simulink model "Quadrotor"  (R2022b)
settings: Solver=FixedStepAuto  StartTime=0.0  StopTime=1000  FixedStep=0.0005  RelTol=1e-3
model workspace (MAT data in the model file):
  b = 0.000142
  g = 9.8
  m = 1
undefined symbols (not defined in the file): Pitch, Roll, X, Y, Yaw, Z
libraries: simulink x12, slpidlib x9, sharedtransform x1, uavutilslib x1, aerolibanim x1
(part 1 of 3)
settings Model: Creator=huawei  LastModifiedBy=Powehi
settings SolverCC: ZeroCrossAlgorithm=Adaptive
settings DebuggingCC: IgnoredZcDiagnostic=none  UnconnectedInputMsg=warning  UnconnectedOutputMsg=warning  UnconnectedLineMsg=warning  SFMachineParentedDataDiag=warning
settings ModelReferenceCC: EnableRefExpFcnMdlSchedulingChecks=on

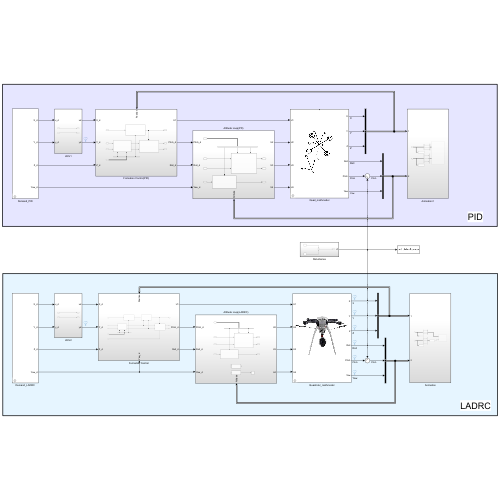
[thumbnail: Simulink's stored preview of the top-level diagram]
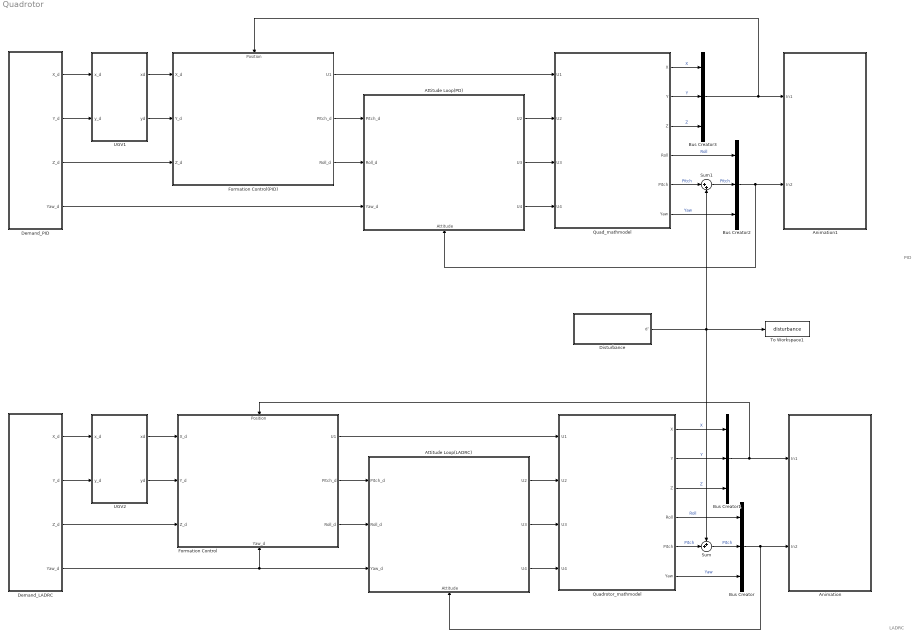
== system Quadrotor ==
  note: PID
  note: LADRC
  Animation : Subsystem
  Animation1 : Subsystem
  Attitude Loop(LADRC) : Subsystem
      settings: PortSchema="{\"entries\":[{\"content\":{\"sides\":[{\"content\":{\"connectorIds\":[\"In1\",\"In2\",\"In3\"]},\"type\":\"ConnectorPlacement.EquallySpacedRectSide\",\"uuid\":\"741c63cb-3193-49ed-b6fe-0554dd8eb38b\"},{\"content\":{\"connectorIds\":[\"Out1\",\"Out2\",\"Out3\"],\"side\":\"RIGHT\"},\"type\":\"ConnectorPlacement.EquallySpacedRectSide\",\"uuid\":\"55d4e1d6-ced0-4d00-88f3-94ecae3eab08\"},{\"content\":{\"connectorIds\":[],\"side\":\"TOP\"},\"type\":\"ConnectorPlacement.EquallySpacedRectSide\",\"uuid\":\"670d5dfa-1a50-4aee-963c-097076b25aa9\"},{\"content\":{\"connectorIds\":[\"In4\"],\"side\":\"BOTTOM\"},\"type\":\"ConnectorPlacement.EquallySpacedRectSide\",\"uuid\":\"461487f9-9010-46f7-8d40-b6bfcadca1df\"}]},\"type\":\"ConnectorPlacement.EquallySpacedConnector\",\"uuid\":\"b0fd4550-2f46-4562-9b6e-a30bcd34312f\"}],\"packageUris\":[\"http://schema.mathworks.com/mf0/Connector/19700101\"],\"version\":\"1.0\"}"
  Attitude Loop(PD) : Subsystem
      settings: PortSchema="{\"entries\":[{\"content\":{\"sides\":[{\"content\":{\"connectorIds\":[\"In1\",\"In2\",\"In3\"]},\"type\":\"ConnectorPlacement.EquallySpacedRectSide\",\"uuid\":\"741c63cb-3193-49ed-b6fe-0554dd8eb38b\"},{\"content\":{\"connectorIds\":[\"Out1\",\"Out2\",\"Out3\"],\"side\":\"RIGHT\"},\"type\":\"ConnectorPlacement.EquallySpacedRectSide\",\"uuid\":\"55d4e1d6-ced0-4d00-88f3-94ecae3eab08\"},{\"content\":{\"connectorIds\":[],\"side\":\"TOP\"},\"type\":\"ConnectorPlacement.EquallySpacedRectSide\",\"uuid\":\"670d5dfa-1a50-4aee-963c-097076b25aa9\"},{\"content\":{\"connectorIds\":[\"In4\"],\"side\":\"BOTTOM\"},\"type\":\"ConnectorPlacement.EquallySpacedRectSide\",\"uuid\":\"461487f9-9010-46f7-8d40-b6bfcadca1df\"}]},\"type\":\"ConnectorPlacement.EquallySpacedConnector\",\"uuid\":\"b0fd4550-2f46-4562-9b6e-a30bcd34312f\"}],\"packageUris\":[\"http://schema.mathworks.com/mf0/Connector/R2020b\"],\"version\":\"1.0\"}"
  Bus Creator : BusCreator  Inputs=Roll,Pitch,Yaw
  Bus Creator1 : BusCreator  Inputs=X,Y,Z
  Bus Creator2 : BusCreator  Inputs=Roll,Pitch,Yaw
  Bus Creator3 : BusCreator  Inputs=X,Y,Z
  Demand_LADRC : Subsystem  mask{s=4}
      mask DialogControl ParameterGroupVar Prompt: 轨迹选择
      mask DialogControl Control8 Prompt: 请输入轨迹序号
      mask DialogControl Container7 Prompt: 展开
      mask DialogControl Control1 Prompt: 1.上升
      mask DialogControl Control2 Prompt: 2.直线
      mask DialogControl Control3 Prompt: 3.环形轨迹
      mask DialogControl Control4 Prompt: 4.螺旋轨迹
      mask DialogControl Control5 Prompt: 5.蝶形轨迹
      mask DialogControl Control7 Prompt: 启动
      mask DialogControl Control7 Callback:
      | clear
      | sim('Quadrotor')
      | figure(1)
      | 
      |   comet3(ans.position(:,1),ans.position(:,2),ans.position(:,end),0.1)%彗星/动图轨迹
      |   title('飞行动态显示图')
      |   grid on
      | 
      | figure(2)
      | subplot(2,2,1)%轨迹线图
      |   plot3(ans.position(:,1),ans.position(:,2),ans.position(:,end),"r",'LineWidth',2) ;%绘制轨迹线图
      |    hold on
      |   plot3(ans.demand(:,1),ans.demand(:,2),ans.demand(:,3),"b--",'LineWidth',2) %绘制输入
      |    hold on
      |    plot3(0,0,0,'g.','markersize',30)%标起始位置
      |    xlabel('X/m');ylabel('Y/m');zlabel('Z/m');%坐标轴名称
      |    legend('飞行轨迹','给定路线')
      |    text(0,0,0,'起始点')
      |    title('飞行轨迹图')
      |    grid on
      | 
      | subplot(2,2,2)%x跟踪对比
      | 
      |    plot(ans.position(:,1),'r','LineWidth',2)%x输出
      |     hold on
      |    plot(ans.demand(:,1),'b--','LineWidth',2)%x给定值
      |     set(gca,'XTick',0:400000:2000000);set(gca,'XTicklabel',{'0','200','400','600','800','1000'})%标定刻度
      |     xlabel('t/s');ylabel('X&Xd');%坐标轴名称
      |     axis([0 inf -1.5 1.5])%坐标范围
      |     legend('x','xd')
      |     title('X坐标跟踪')
      |     grid on%网格
      | 
      | subplot(2,2,3)%y跟踪对比
      | 
      |    plot(ans.position(:,2),'r','LineWidth',2)
      |     hold on
      |    plot(ans.demand(:,2),'b--','LineWidth',2)
      |     set(gca,'XTick',0:400000:2000000);set(gca,'XTicklabel',{'0','200','400','600','800','1000'})
      |     xlabel('t/s');ylabel('Y&Yd');
      |     axis([0 inf -1.5 1.5])
      |     legend('y','yd')
      |     title('Y坐标跟踪')
      |     grid on
      | subplot(2,2,4)%z跟踪对比
      | 
      |    plot(ans.position(:,end),'r','LineWidth',2)
      |     hold on
      |    plot(ans.demand(:,3),'b--','LineWidth',2)
      |     set(gca,'XTick',0:400000:2000000);set(gca,'XTicklabel',{'0','200','400','600','800','1000'})
      |     xlabel('t/s');ylabel('Z&Zd');
      |     axis([0 inf 0 7])
      |     legend('z','zd')
      |     title('Z坐标跟踪')
      |     grid on
  Demand_PID : Subsystem  mask{s=4}
      mask DialogControl ParameterGroupVar Prompt: 轨迹选择
      mask DialogControl Control8 Prompt: 请输入轨迹序号
      mask DialogControl Container7 Prompt: 展开
      mask DialogControl Control1 Prompt: 1.上升
      mask DialogControl Control2 Prompt: 2.直线
      mask DialogControl Control3 Prompt: 3.环形轨迹
      mask DialogControl Control4 Prompt: 4.螺旋轨迹
      mask DialogControl Control5 Prompt: 5.蝶形轨迹
      mask DialogControl Control7 Prompt: 启动
      mask DialogControl Control7 Callback:
      | clear
      | sim('Quadrotor_PID_final')
      | figure(1)
      | 
      |   comet3(ans.position(:,1),ans.position(:,2),ans.position(:,end),0.1)%彗星/动图轨迹
      |   title('飞行动态显示图')
      |   grid on
      | 
      | figure(2)
      | subplot(2,2,1)%轨迹线图
      |   plot3(ans.position(:,1),ans.position(:,2),ans.position(:,end),"r",'LineWidth',2) ;%绘制轨迹线图
      |    hold on
      |   plot3(ans.demand(:,1),ans.demand(:,2),ans.demand(:,3),"b--",'LineWidth',2) %绘制输入
      |    hold on
      |    plot3(0,0,0,'g.','markersize',30)%标起始位置
      |    xlabel('X/m');ylabel('Y/m');zlabel('Z/m');%坐标轴名称
      |    legend('飞行轨迹','给定路线')
      |    text(0,0,0,'起始点')
      |    title('飞行轨迹图')
      |    grid on
      | 
      | subplot(2,2,2)%x跟踪对比
      | 
      |    plot(ans.position(:,1),'r','LineWidth',2)%x输出
      |     hold on
      |    plot(ans.demand(:,1),'b--','LineWidth',2)%x给定值
      |     set(gca,'XTick',0:1200:6000);set(gca,'XTicklabel',{'0','200','400','600','800','1000'})%标定刻度
      |     xlabel('t/s');ylabel('X&Xd');%坐标轴名称
      |     axis([0 inf -1.5 1.5])%坐标范围
      |     legend('x','xd')
      |     title('X坐标跟踪')
      |     grid on%网格
      | 
      | subplot(2,2,3)%y跟踪对比
      | 
      |    plot(ans.position(:,2),'r','LineWidth',2)
      |     hold on
      |    plot(ans.demand(:,2),'b--','LineWidth',2)
      |     set(gca,'XTick',0:1200:6000);set(gca,'XTicklabel',{'0','200','400','600','800','1000'})
      |     xlabel('t/s');ylabel('Y&Yd');
      |     axis([0 inf -1.5 1.5])
      |     legend('y','yd')
      |     title('Y坐标跟踪')
      |     grid on
      | subplot(2,2,4)%z跟踪对比
      | 
      |    plot(ans.position(:,end),'r','LineWidth',2)
      |     hold on
      |    plot(ans.demand(:,3),'b--','LineWidth',2)
      |     set(gca,'XTick',0:1200:6000);set(gca,'XTicklabel',{'0','200','400','600','800','1000'})
      |     xlabel('t/s');ylabel('Z&Zd');
      |     axis([0 inf 0 7])
      |     legend('z','zd')
      |     title('Z坐标跟踪')
      |     grid on
  Disturbance : Subsystem
  Formation Control : Subsystem
      settings: PortSchema="{\"entries\":[{\"content\":{\"sides\":[{\"content\":{\"connectorIds\":[\"In1\",\"In2\",\"In3\"]},\"type\":\"ConnectorPlacement.EquallySpacedRectSide\",\"uuid\":\"741c63cb-3193-49ed-b6fe-0554dd8eb38b\"},{\"content\":{\"connectorIds\":[\"Out1\",\"Out2\",\"Out3\"],\"side\":\"RIGHT\"},\"type\":\"ConnectorPlacement.EquallySpacedRectSide\",\"uuid\":\"55d4e1d6-ced0-4d00-88f3-94ecae3eab08\"},{\"content\":{\"connectorIds\":[\"In4\"],\"side\":\"TOP\"},\"type\":\"ConnectorPlacement.EquallySpacedRectSide\",\"uuid\":\"670d5dfa-1a50-4aee-963c-097076b25aa9\"},{\"content\":{\"connectorIds\":[\"In5\"],\"side\":\"BOTTOM\"},\"type\":\"ConnectorPlacement.EquallySpacedRectSide\",\"uuid\":\"31dc6e32-e4ae-4a63-8318-e80959689dd0\"}]},\"type\":\"ConnectorPlacement.EquallySpacedConnector\",\"uuid\":\"b0fd4550-2f46-4562-9b6e-a30bcd34312f\"}],\"packageUris\":[\"http://schema.mathworks.com/mf0/Connector/R2020b\"],\"version\":\"1.0\"}"
  Formation Control(PID) : Subsystem
      settings: PortSchema="{\"entries\":[{\"content\":{\"sides\":[{\"content\":{\"connectorIds\":[\"In1\",\"In2\",\"In3\"]},\"type\":\"ConnectorPlacement.EquallySpacedRectSide\",\"uuid\":\"741c63cb-3193-49ed-b6fe-0554dd8eb38b\"},{\"content\":{\"connectorIds\":[\"Out1\",\"Out2\",\"Out3\"],\"side\":\"RIGHT\"},\"type\":\"ConnectorPlacement.EquallySpacedRectSide\",\"uuid\":\"55d4e1d6-ced0-4d00-88f3-94ecae3eab08\"},{\"content\":{\"connectorIds\":[\"In4\"],\"side\":\"TOP\"},\"type\":\"ConnectorPlacement.EquallySpacedRectSide\",\"uuid\":\"670d5dfa-1a50-4aee-963c-097076b25aa9\"},{\"content\":{\"connectorIds\":[],\"side\":\"BOTTOM\"},\"type\":\"ConnectorPlacement.EquallySpacedRectSide\",\"uuid\":\"31dc6e32-e4ae-4a63-8318-e80959689dd0\"}]},\"type\":\"ConnectorPlacement.EquallySpacedConnector\",\"uuid\":\"b0fd4550-2f46-4562-9b6e-a30bcd34312f\"}],\"packageUris\":[\"http://schema.mathworks.com/mf0/Connector/R2020b\"],\"version\":\"1.0\"}"
  Quad_mathmodel : Subsystem  mask{m=1, L=0.24, b=1.42e-4, d=6.21e-5, g=9.8, Ix=8.1e-3, Iy=8.1e-3, Iz=12.4e-3, Jtp=7.24e-5}
      mask DialogControl ParameterGroupVar Prompt: 四旋翼飞行器参数设置
      mask DialogControl Container10 Prompt: 飞行器质量(kg)
      mask DialogControl Container11 Prompt: 质心到电机中心轴距(m)
      mask DialogControl Container16 Prompt: 升力系数
      mask DialogControl Container15 Prompt: 阻力系数
      mask DialogControl Container14 Prompt: 重力加速度
      mask DialogControl Container13 Prompt: 绕X轴转动惯量
      mask DialogControl Container12 Prompt: 绕Y轴转动惯量
      mask DialogControl Container17 Prompt: 绕Z轴转动惯量
      mask DialogControl Container18 Prompt: 机体绕转轴的总转动惯量（可忽略）
      mask Display: image('$imagefile'); % Use "Edit Image" on toolstrip to change.
  Quadrotor_mathmodel : Subsystem  mask{m=1, L=0.24, b=1.42e-4, d=6.21e-5, g=9.8, Ix=8.1e-3, Iy=8.1e-3, Iz=12.4e-3, Jtp=7.24e-5}
      mask DialogControl ParameterGroupVar Prompt: 四旋翼飞行器参数设置
      mask DialogControl Container10 Prompt: 飞行器质量(kg)
      mask DialogControl Container11 Prompt: 质心到电机中心轴距(m)
      mask DialogControl Container16 Prompt: 升力系数
      mask DialogControl Container15 Prompt: 阻力系数
      mask DialogControl Container14 Prompt: 重力加速度
      mask DialogControl Container13 Prompt: 绕X轴转动惯量
      mask DialogControl Container12 Prompt: 绕Y轴转动惯量
      mask DialogControl Container17 Prompt: 绕Z轴转动惯量
      mask DialogControl Container18 Prompt: 机体绕转轴的总转动惯量（可忽略）
      mask Display: image('$imagefile'); % Use "Edit Image" on toolstrip to change.
  Sum : Sum  Inputs=++|
  Sum1 : Sum  Inputs=|++
  To Workspace1 : ToWorkspace  VariableName=disturbance  SampleTime=-1
  UGV1 : Subsystem
  UGV2 : Subsystem
  wires:
  Quadrotor_mathmodel/6(Yaw) -> Bus Creator/3  "Yaw"
  Quadrotor_mathmodel/3(Z) -> Bus Creator1/3  "Z"
  Formation Control/1(U1) -> Quadrotor_mathmodel/1(U1)
  Formation Control/2(Pitch_d) -> Attitude Loop(LADRC)/1(Pitch_d)
  Formation Control/3(Roll_d) -> Attitude Loop(LADRC)/2(Roll_d)
  Attitude Loop(LADRC)/3(U4) -> Quadrotor_mathmodel/4(U4)
  Attitude Loop(LADRC)/1(U2) -> Quadrotor_mathmodel/2(U2)
  Attitude Loop(LADRC)/2(U3) -> Quadrotor_mathmodel/3(U3)
  Quadrotor_mathmodel/4(Roll) -> Bus Creator/1  "Roll"
  Bus Creator1/1 -> Animation/1(In1), Formation Control/4(Position)
  Bus Creator/1 -> Attitude Loop(LADRC)/4(Attitude), Animation/2(In2)
  Demand_LADRC/1(X_d) -> UGV2/1(x_d)
  UGV2/1(xd) -> Formation Control/1(X_d)
  Demand_LADRC/2(Y_d) -> UGV2/2(y_d)
  UGV2/2(yd) -> Formation Control/2(Y_d)
  Demand_LADRC/3(Z_d) -> Formation Control/3(Z_d)
  Demand_LADRC/4(Yaw_d) -> Formation Control/5(Yaw_d), Attitude Loop(LADRC)/3(Yaw_d)
  Quadrotor_mathmodel/1(X) -> Bus Creator1/1  "X"
  Quadrotor_mathmodel/2(Y) -> Bus Creator1/2  "Y"
  Sum/1 -> Bus Creator/2  "Pitch"
  Quadrotor_mathmodel/5(Pitch) -> Sum/2  "Pitch"
  Disturbance/1(d') -> To Workspace1/1, Sum1/2, Sum/1
  Demand_PID/3(Z_d) -> Formation Control(PID)/3(Z_d)
  Quad_mathmodel/1(X) -> Bus Creator3/1  "X"
  Demand_PID/4(Yaw_d) -> Attitude Loop(PD)/3(Yaw_d)
  Attitude Loop(PD)/1(U2) -> Quad_mathmodel/2(U2)
  Quad_mathmodel/3(Z) -> Bus Creator3/3  "Z"
  Attitude Loop(PD)/3(U4) -> Quad_mathmodel/4(U4)
  Attitude Loop(PD)/2(U3) -> Quad_mathmodel/3(U3)
  Formation Control(PID)/3(Roll_d) -> Attitude Loop(PD)/2(Roll_d)
  Bus Creator2/1 -> Attitude Loop(PD)/4(Attitude), Animation1/2(In2)
  Quad_mathmodel/2(Y) -> Bus Creator3/2  "Y"
  Quad_mathmodel/4(Roll) -> Bus Creator2/1  "Roll"
  Formation Control(PID)/2(Pitch_d) -> Attitude Loop(PD)/1(Pitch_d)
  Formation Control(PID)/1(U1) -> Quad_mathmodel/1(U1)
  Bus Creator3/1 -> Formation Control(PID)/4(Position), Animation1/1(In1)
  Quad_mathmodel/6(Yaw) -> Bus Creator2/3  "Yaw"
  Sum1/1 -> Bus Creator2/2  "Pitch"
  Quad_mathmodel/5(Pitch) -> Sum1/1  "Pitch"
  UGV1/1(xd) -> Formation Control(PID)/1(X_d)
  UGV1/2(yd) -> Formation Control(PID)/2(Y_d)
  Demand_PID/2(Y_d) -> UGV1/2(y_d)
  Demand_PID/1(X_d) -> UGV1/1(x_d)

== system Quadrotor/Animation ==
  In1 : Inport
  In2 : Inport  Port=2
  Bus Creator2 : BusCreator  Inputs=3
  Bus Creator3 : BusCreator  Inputs=3
  Bus Selector : BusSelector  OutputSignals=X,Y,Z
  Bus Selector1 : BusSelector  OutputSignals=Roll,Pitch,Yaw
  Rotation Angles to Quaternions : sharedtransform/Rotation Angles to Quaternions  rotationOrder=XYZ  aMode=aMode
  To Workspace : ToWorkspace  VariableName=position1  SampleTime=-1
  To Workspace1 : ToWorkspace  VariableName=attitude1  SampleTime=-1
  UAV Animation : uavutilslib/UAV Animation  Commented=on  UAVType=Multirotor  UAVSize=0.1  InertialZDirection=Up  SampleTime=-1
  wires:
  In1/1 -> Bus Selector/1, To Workspace/1
  Bus Selector1/1 -> Bus Creator2/1  "<Roll>"
  In2/1 -> To Workspace1/1, Bus Selector1/1
  Bus Selector/2 -> Bus Creator3/2  "<Y>"
  Bus Selector1/2 -> Bus Creator2/2  "<Pitch>"
  Bus Selector/3 -> Bus Creator3/3  "<Z>"
  Bus Selector/1 -> Bus Creator3/1  "<X>"
  Bus Selector1/3 -> Bus Creator2/3  "<Yaw>"
  Bus Creator2/1 -> Rotation Angles to Quaternions/1
  Rotation Angles to Quaternions/1 -> UAV Animation/2
  Bus Creator3/1 -> UAV Animation/1

== system Quadrotor/Animation1 ==
  In1 : Inport
  In2 : Inport  Port=2
  6DoF Animation : aerolibanim/6DoF Animation  Commented=on  u1=[-2 2 -2 2 -4 0]  u2=0.1  u3=0.5  u4=[0 0 4]  u5=Fixed position  u6=[40 0 -0.5]  u7=7  u8=on
  Bus Creator2 : BusCreator  Inputs=3
  Bus Creator3 : BusCreator  Inputs=3
  Bus Selector : BusSelector  OutputSignals=X,Y,Z
  Bus Selector1 : BusSelector  OutputSignals=Roll,Pitch,Yaw
  To Workspace : ToWorkspace  VariableName=position  SampleTime=-1
  To Workspace1 : ToWorkspace  VariableName=attitude  SampleTime=-1
  wires:
  In1/1 -> Bus Selector/1, To Workspace/1
  Bus Selector1/1 -> Bus Creator2/1  "<Roll>"
  In2/1 -> To Workspace1/1, Bus Selector1/1
  Bus Selector/2 -> Bus Creator3/2  "<Y>"
  Bus Selector1/2 -> Bus Creator2/2  "<Pitch>"
  Bus Creator2/1 -> 6DoF Animation/2
  Bus Selector/3 -> Bus Creator3/3  "<Z>"
  Bus Creator3/1 -> 6DoF Animation/1
  Bus Selector/1 -> Bus Creator3/1  "<X>"
  Bus Selector1/3 -> Bus Creator2/3  "<Yaw>"

== system Quadrotor/Attitude Loop(LADRC) ==
  Pitch_d : Inport
  Roll_d : Inport  Port=2
  Yaw_d : Inport  Port=3
  Attitude : Inport  Port=4
  Bus Selector : BusSelector  OutputSignals=Yaw,Pitch,Roll
  LADRC : Subsystem  mask{h=0.0005, r=100, beta01=100, beta02=200, beta03=300, kp1=5, kp2=5, b=1}
      mask DialogControl ParameterGroupVar Prompt: 四旋翼参数
      mask DialogControl Container3 Prompt: 步长
      mask DialogControl Container4 Prompt: 跟踪速度
      mask DialogControl Container5 Prompt: 增益
      mask DialogControl Container6 Prompt: 系统增益
  LADRC1 : Subsystem  mask{h=0.0005, r=100, beta01=100, beta02=200, beta03=300, kp1=5, kp2=5, b=1}
      mask DialogControl ParameterGroupVar Prompt: 四旋翼参数
      mask DialogControl Container3 Prompt: 步长
      mask DialogControl Container4 Prompt: 跟踪速度
      mask DialogControl Container5 Prompt: 增益
      mask DialogControl Container6 Prompt: 系统增益
  P&R : Subsystem
      settings: PortSchema="{\"entries\":[{\"content\":{\"sides\":[{\"content\":{\"connectorIds\":[\"In1\",\"In2\"]},\"type\":\"ConnectorPlacement.EquallySpacedRectSide\",\"uuid\":\"5a168f57-9082-4ef9-b723-ec42d235f15b\"},{\"content\":{\"connectorIds\":[\"Out1\",\"Out2\"],\"side\":\"RIGHT\"},\"type\":\"ConnectorPlacement.EquallySpacedRectSide\",\"uuid\":\"1b4dc671-5a32-4537-87d8-64b7817d412d\"},{\"content\":{\"connectorIds\":[\"In3\",\"In4\"],\"side\":\"TOP\"},\"type\":\"ConnectorPlacement.EquallySpacedRectSide\",\"uuid\":\"3d489923-4a97-462b-9fd9-288b2bf2a159\"}]},\"type\":\"ConnectorPlacement.EquallySpacedConnector\",\"uuid\":\"91228c47-fce9-4c1d-8a3a-204dc80f90dd\"}],\"packageUris\":[\"http://schema.mathworks.com/mf0/Connector/R2020b\"],\"version\":\"1.0\"}"
  Scope : Scope
  yaw : Subsystem
      settings: PortSchema="{\"entries\":[{\"content\":{\"sides\":[{\"content\":{\"connectorIds\":[\"In1\"]},\"type\":\"ConnectorPlacement.EquallySpacedRectSide\",\"uuid\":\"a7b1533a-1266-40d5-b52c-012082b26468\"},{\"content\":{\"connectorIds\":[\"Out1\"],\"side\":\"RIGHT\"},\"type\":\"ConnectorPlacement.EquallySpacedRectSide\",\"uuid\":\"b4620233-0e85-40ae-9738-c29ba1209ef5\"},{\"content\":{\"connectorIds\":[\"In2\"],\"side\":\"TOP\"},\"type\":\"ConnectorPlacement.EquallySpacedRectSide\",\"uuid\":\"ab9c222c-25de-47f6-b54f-342fd8d0321b\"},{\"content\":{\"connectorIds\":[],\"side\":\"BOTTOM\"},\"type\":\"ConnectorPlacement.EquallySpacedRectSide\",\"uuid\":\"5eacbb93-3d5d-4d57-aaef-fda87c8b1f96\"}]},\"type\":\"ConnectorPlacement.EquallySpacedConnector\",\"uuid\":\"8cc1c8e9-c992-4e05-8575-ab9d3ec9e6a4\"}],\"packageUris\":[\"http://schema.mathworks.com/mf0/Connector/R2020b\"],\"version\":\"1.0\"}"
  U2 : Outport
  U3 : Outport  Port=2
  U4 : Outport  Port=3
  wires:
  Bus Selector/2 -> P&R/3(Pitch)  "<Pitch>"
  Roll_d/1 -> P&R/2(Roll_d)
  yaw/1(U4) -> U4/1
  Attitude/1 -> Bus Selector/1
  Bus Selector/3 -> P&R/4(Roll)  "<Roll>"
  Pitch_d/1 -> P&R/1(Pitch_d)
  Bus Selector/1 -> yaw/2(Yaw)  "<Yaw>"
  P&R/2(U2) -> U2/1
  P&R/1(U3) -> U3/1
  Yaw_d/1 -> yaw/1(Yaw_d)
  LADRC/1(y) -> Scope/1

== system Quadrotor/Attitude Loop(PD) ==
  Pitch_d : Inport
  Roll_d : Inport  Port=2
  Yaw_d : Inport  Port=3
  Attitude : Inport  Port=4
  Bus Selector : BusSelector  OutputSignals=Yaw,Pitch,Roll
  P&R : Subsystem
      settings: PortSchema="{\"entries\":[{\"content\":{\"sides\":[{\"content\":{\"connectorIds\":[\"In1\",\"In2\"]},\"type\":\"ConnectorPlacement.EquallySpacedRectSide\",\"uuid\":\"5a168f57-9082-4ef9-b723-ec42d235f15b\"},{\"content\":{\"connectorIds\":[\"Out1\",\"Out2\"],\"side\":\"RIGHT\"},\"type\":\"ConnectorPlacement.EquallySpacedRectSide\",\"uuid\":\"1b4dc671-5a32-4537-87d8-64b7817d412d\"},{\"content\":{\"connectorIds\":[\"In3\",\"In4\"],\"side\":\"TOP\"},\"type\":\"ConnectorPlacement.EquallySpacedRectSide\",\"uuid\":\"3d489923-4a97-462b-9fd9-288b2bf2a159\"}]},\"type\":\"ConnectorPlacement.EquallySpacedConnector\",\"uuid\":\"91228c47-fce9-4c1d-8a3a-204dc80f90dd\"}],\"packageUris\":[\"http://schema.mathworks.com/mf0/Connector/R2020b\"],\"version\":\"1.0\"}"
  yaw : Subsystem
      settings: PortSchema="{\"entries\":[{\"content\":{\"sides\":[{\"content\":{\"connectorIds\":[\"In1\"]},\"type\":\"ConnectorPlacement.EquallySpacedRectSide\",\"uuid\":\"a7b1533a-1266-40d5-b52c-012082b26468\"},{\"content\":{\"connectorIds\":[\"Out1\"],\"side\":\"RIGHT\"},\"type\":\"ConnectorPlacement.EquallySpacedRectSide\",\"uuid\":\"b4620233-0e85-40ae-9738-c29ba1209ef5\"},{\"content\":{\"connectorIds\":[\"In2\"],\"side\":\"TOP\"},\"type\":\"ConnectorPlacement.EquallySpacedRectSide\",\"uuid\":\"ab9c222c-25de-47f6-b54f-342fd8d0321b\"},{\"content\":{\"connectorIds\":[],\"side\":\"BOTTOM\"},\"type\":\"ConnectorPlacement.EquallySpacedRectSide\",\"uuid\":\"5eacbb93-3d5d-4d57-aaef-fda87c8b1f96\"}]},\"type\":\"ConnectorPlacement.EquallySpacedConnector\",\"uuid\":\"8cc1c8e9-c992-4e05-8575-ab9d3ec9e6a4\"}],\"packageUris\":[\"http://schema.mathworks.com/mf0/Connector/R2020b\"],\"version\":\"1.0\"}"
  U2 : Outport
  U3 : Outport  Port=2
  U4 : Outport  Port=3
  wires:
  Bus Selector/2 -> P&R/3(Pitch)  "<Pitch>"
  Roll_d/1 -> P&R/2(Roll_d)
  yaw/1(U4) -> U4/1
  Attitude/1 -> Bus Selector/1
  Bus Selector/3 -> P&R/4(Roll)  "<Roll>"
  Pitch_d/1 -> P&R/1(Pitch_d)
  Bus Selector/1 -> yaw/2(Yaw)  "<Yaw>"
  P&R/2(U2) -> U2/1
  P&R/1(U3) -> U3/1
  Yaw_d/1 -> yaw/1(Yaw_d)

== system Quadrotor/Demand_LADRC ==
  Multiport Switch : MultiPortSwitch  Inputs=6  SaturateOnIntegerOverflow=off  InputSameDT=off
  generate : Subsystem
  out : Subsystem
  select number : Constant  Value=s
  X_d : Outport
  Y_d : Outport  Port=2
  Z_d : Outport  Port=3
  Yaw_d : Outport  Port=4
  wires:
  out/1(X_d) -> X_d/1
  out/2(Y_d) -> Y_d/1
  out/3(Z_d) -> Z_d/1
  out/4(Yaw_d) -> Yaw_d/1
  Multiport Switch/1 -> out/1(In1)
  generate/1(up) -> Multiport Switch/2
  generate/2(ramp) -> Multiport Switch/3
  generate/3(circle) -> Multiport Switch/4
  generate/4(screw) -> Multiport Switch/5
  generate/5(butterfiy) -> Multiport Switch/6
  select number/1 -> Multiport Switch/1
  generate/6(steady) -> Multiport Switch/7

== system Quadrotor/Demand_PID ==
  Multiport Switch : MultiPortSwitch  Inputs=6  SaturateOnIntegerOverflow=off  InputSameDT=off
  generate : Subsystem
  out : Subsystem
  select number : Constant  Value=s
  X_d : Outport
  Y_d : Outport  Port=2
  Z_d : Outport  Port=3
  Yaw_d : Outport  Port=4
  wires:
  out/1(X_d) -> X_d/1
  out/2(Y_d) -> Y_d/1
  out/3(Z_d) -> Z_d/1
  out/4(Yaw_d) -> Yaw_d/1
  Multiport Switch/1 -> out/1(In1)
  generate/1(up) -> Multiport Switch/2
  generate/2(ramp) -> Multiport Switch/3
  generate/3(circle) -> Multiport Switch/4
  generate/4(screw) -> Multiport Switch/5
  generate/5(butterfiy) -> Multiport Switch/6
  select number/1 -> Multiport Switch/1
  generate/6(steady) -> Multiport Switch/7

== system Quadrotor/Disturbance ==
  Step : Step  Time=20  After=0.01  SampleTime=0.0005
  Step1 : Step  Time=22  After=-0.01  SampleTime=0.0005
  Sum : Sum
  d' : Outport
  wires:
  Step/1 -> Sum/1
  Step1/1 -> Sum/2
  Sum/1 -> d'/1

== system Quadrotor/Formation Control ==
  X_d : Inport
  Y_d : Inport  Port=2
  Z_d : Inport  Port=3
  Position : Inport  Port=4
  Yaw_d : Inport  Port=5
  Bus Selector1 : BusSelector  OutputSignals=X,Y,Z
  height : Subsystem
      settings: PortSchema="{\"entries\":[{\"content\":{\"sides\":[{\"content\":{\"connectorIds\":[\"In1\"]},\"type\":\"ConnectorPlacement.EquallySpacedRectSide\",\"uuid\":\"a7b1533a-1266-40d5-b52c-012082b26468\"},{\"content\":{\"connectorIds\":[\"Out1\"],\"side\":\"RIGHT\"},\"type\":\"ConnectorPlacement.EquallySpacedRectSide\",\"uuid\":\"b4620233-0e85-40ae-9738-c29ba1209ef5\"},{\"content\":{\"connectorIds\":[],\"side\":\"TOP\"},\"type\":\"ConnectorPlacement.EquallySpacedRectSide\",\"uuid\":\"ab9c222c-25de-47f6-b54f-342fd8d0321b\"},{\"content\":{\"connectorIds\":[\"In2\"],\"side\":\"BOTTOM\"},\"type\":\"ConnectorPlacement.EquallySpacedRectSide\",\"uuid\":\"c0ec5864-a2e3-4dc9-86df-2e8e31dc698f\"}]},\"type\":\"ConnectorPlacement.EquallySpacedConnector\",\"uuid\":\"8cc1c8e9-c992-4e05-8575-ab9d3ec9e6a4\"}],\"packageUris\":[\"http://schema.mathworks.com/mf0/Connector/R2020b\"],\"version\":\"1.0\"}"
  "location " : Subsystem
      settings: PortSchema="{\"entries\":[{\"content\":{\"sides\":[{\"content\":{\"connectorIds\":[\"In1\",\"In2\"]},\"type\":\"ConnectorPlacement.EquallySpacedRectSide\",\"uuid\":\"5a168f57-9082-4ef9-b723-ec42d235f15b\"},{\"content\":{\"connectorIds\":[\"Out1\",\"Out2\"],\"side\":\"RIGHT\"},\"type\":\"ConnectorPlacement.EquallySpacedRectSide\",\"uuid\":\"1b4dc671-5a32-4537-87d8-64b7817d412d\"},{\"content\":{\"connectorIds\":[],\"side\":\"TOP\"},\"type\":\"ConnectorPlacement.EquallySpacedRectSide\",\"uuid\":\"3d489923-4a97-462b-9fd9-288b2bf2a159\"},{\"content\":{\"connectorIds\":[\"In3\",\"In4\"],\"side\":\"BOTTOM\"},\"type\":\"ConnectorPlacement.EquallySpacedRectSide\",\"uuid\":\"ca455ebd-18aa-4cdd-b9a1-332337147b86\"}]},\"type\":\"ConnectorPlacement.EquallySpacedConnector\",\"uuid\":\"91228c47-fce9-4c1d-8a3a-204dc80f90dd\"}],\"packageUris\":[\"http://schema.mathworks.com/mf0/Connector/R2020b\"],\"version\":\"1.0\"}"
  operation : Subsystem
      settings: PortSchema="{\"entries\":[{\"content\":{\"sides\":[{\"content\":{\"connectorIds\":[\"In1\",\"In2\"]},\"type\":\"ConnectorPlacement.EquallySpacedRectSide\",\"uuid\":\"7b5ff4eb-d8d0-4c09-9af3-42040e275879\"},{\"content\":{\"connectorIds\":[\"Out1\",\"Out2\"],\"side\":\"RIGHT\"},\"type\":\"ConnectorPlacement.EquallySpacedRectSide\",\"uuid\":\"8346582f-6666-4076-82d0-a237d0151848\"},{\"content\":{\"connectorIds\":[\"In3\"],\"side\":\"TOP\"},\"type\":\"ConnectorPlacement.EquallySpacedRectSide\",\"uuid\":\"392c211c-fa44-4e3a-adf5-1ced3bd87e05\"},{\"content\":{\"connectorIds\":[\"In4\"],\"side\":\"BOTTOM\"},\"type\":\"ConnectorPlacement.EquallySpacedRectSide\",\"uuid\":\"3de96f84-30de-4416-984d-9bfcd650e458\"}]},\"type\":\"ConnectorPlacement.EquallySpacedConnector\",\"uuid\":\"5d751e66-253e-464d-b7a7-9553a5bc15c8\"}],\"packageUris\":[\"http://schema.mathworks.com/mf0/Connector/R2020b\"],\"version\":\"1.0\"}"
  sum : Subsystem
      settings: PortSchema="{\"entries\":[{\"content\":{\"sides\":[{\"content\":{\"connectorIds\":[\"In1\"]},\"type\":\"ConnectorPlacement.EquallySpacedRectSide\",\"uuid\":\"a7b1533a-1266-40d5-b52c-012082b26468\"},{\"content\":{\"connectorIds\":[\"Out1\"],\"side\":\"RIGHT\"},\"type\":\"ConnectorPlacement.EquallySpacedRectSide\",\"uuid\":\"b4620233-0e85-40ae-9738-c29ba1209ef5\"},{\"content\":{\"connectorIds\":[],\"side\":\"TOP\"},\"type\":\"ConnectorPlacement.EquallySpacedRectSide\",\"uuid\":\"ab9c222c-25de-47f6-b54f-342fd8d0321b\"},{\"content\":{\"connectorIds\":[\"In2\",\"In3\"],\"side\":\"BOTTOM\"},\"type\":\"ConnectorPlacement.EquallySpacedRectSide\",\"uuid\":\"c0ec5864-a2e3-4dc9-86df-2e8e31dc698f\"}]},\"type\":\"ConnectorPlacement.EquallySpacedConnector\",\"uuid\":\"8cc1c8e9-c992-4e05-8575-ab9d3ec9e6a4\"}],\"packageUris\":[\"http://schema.mathworks.com/mf0/Connector/R2020b\"],\"version\":\"1.0\"}"
  U1 : Outport
  Pitch_d : Outport  Port=2
  Roll_d : Outport  Port=3
  wires:
  "location "/1(X') -> sum/2(Ux), operation/1(X')
  Bus Selector1/3 -> height/2(Z)  "<Z>"
  Bus Selector1/2 -> "location "/4(Y)  "<Y>"
  Z_d/1 -> height/1(Z_d)
  Bus Selector1/1 -> "location "/3(X)  "<X>"
  Position/1 -> Bus Selector1/1
  "location "/2(Y') -> sum/3(Uy), operation/2(Y')
  operation/2(Roll_d) -> Roll_d/1
  X_d/1 -> "location "/1(X_d)
  Y_d/1 -> "location "/2(Y_d)
  operation/1(Pitch_d) -> Pitch_d/1
  Yaw_d/1 -> operation/4(Yaw_d)
  height/1(Uz+g) -> sum/1(Uz+g)
  sum/1(U1) -> operation/3(U1), U1/1

== system Quadrotor/Formation Control(PID) ==
  X_d : Inport
  Y_d : Inport  Port=2
  Z_d : Inport  Port=3
  Position : Inport  Port=4
  Bus Selector1 : BusSelector  OutputSignals=X,Y,Z
  height : Subsystem
      settings: PortSchema="{\"entries\":[{\"content\":{\"sides\":[{\"content\":{\"connectorIds\":[\"In1\"]},\"type\":\"ConnectorPlacement.EquallySpacedRectSide\",\"uuid\":\"a7b1533a-1266-40d5-b52c-012082b26468\"},{\"content\":{\"connectorIds\":[\"Out1\"],\"side\":\"RIGHT\"},\"type\":\"ConnectorPlacement.EquallySpacedRectSide\",\"uuid\":\"b4620233-0e85-40ae-9738-c29ba1209ef5\"},{\"content\":{\"connectorIds\":[],\"side\":\"TOP\"},\"type\":\"ConnectorPlacement.EquallySpacedRectSide\",\"uuid\":\"ab9c222c-25de-47f6-b54f-342fd8d0321b\"},{\"content\":{\"connectorIds\":[\"In2\"],\"side\":\"BOTTOM\"},\"type\":\"ConnectorPlacement.EquallySpacedRectSide\",\"uuid\":\"c0ec5864-a2e3-4dc9-86df-2e8e31dc698f\"}]},\"type\":\"ConnectorPlacement.EquallySpacedConnector\",\"uuid\":\"8cc1c8e9-c992-4e05-8575-ab9d3ec9e6a4\"}],\"packageUris\":[\"http://schema.mathworks.com/mf0/Connector/R2020b\"],\"version\":\"1.0\"}"
  "location " : Subsystem
      settings: PortSchema="{\"entries\":[{\"content\":{\"sides\":[{\"content\":{\"connectorIds\":[\"In1\",\"In2\"]},\"type\":\"ConnectorPlacement.EquallySpacedRectSide\",\"uuid\":\"5a168f57-9082-4ef9-b723-ec42d235f15b\"},{\"content\":{\"connectorIds\":[\"Out1\",\"Out2\"],\"side\":\"RIGHT\"},\"type\":\"ConnectorPlacement.EquallySpacedRectSide\",\"uuid\":\"1b4dc671-5a32-4537-87d8-64b7817d412d\"},{\"content\":{\"connectorIds\":[],\"side\":\"TOP\"},\"type\":\"ConnectorPlacement.EquallySpacedRectSide\",\"uuid\":\"3d489923-4a97-462b-9fd9-288b2bf2a159\"},{\"content\":{\"connectorIds\":[\"In3\",\"In4\"],\"side\":\"BOTTOM\"},\"type\":\"ConnectorPlacement.EquallySpacedRectSide\",\"uuid\":\"ca455ebd-18aa-4cdd-b9a1-332337147b86\"}]},\"type\":\"ConnectorPlacement.EquallySpacedConnector\",\"uuid\":\"91228c47-fce9-4c1d-8a3a-204dc80f90dd\"}],\"packageUris\":[\"http://schema.mathworks.com/mf0/Connector/R2020b\"],\"version\":\"1.0\"}"
  operation : Subsystem
      settings: PortSchema="{\"entries\":[{\"content\":{\"sides\":[{\"content\":{\"connectorIds\":[\"In1\",\"In2\"]},\"type\":\"ConnectorPlacement.EquallySpacedRectSide\",\"uuid\":\"7b5ff4eb-d8d0-4c09-9af3-42040e275879\"},{\"content\":{\"connectorIds\":[\"Out1\",\"Out2\"],\"side\":\"RIGHT\"},\"type\":\"ConnectorPlacement.EquallySpacedRectSide\",\"uuid\":\"8346582f-6666-4076-82d0-a237d0151848\"},{\"content\":{\"connectorIds\":[\"In3\"],\"side\":\"TOP\"},\"type\":\"ConnectorPlacement.EquallySpacedRectSide\",\"uuid\":\"392c211c-fa44-4e3a-adf5-1ced3bd87e05\"}]},\"type\":\"ConnectorPlacement.EquallySpacedConnector\",\"uuid\":\"5d751e66-253e-464d-b7a7-9553a5bc15c8\"}],\"packageUris\":[\"http://schema.mathworks.com/mf0/Connector/R2020b\"],\"version\":\"1.0\"}"
  U1 : Outport
  Pitch_d : Outport  Port=2
  Roll_d : Outport  Port=3
  wires:
  "location "/1(X') -> operation/1(X')
  Bus Selector1/3 -> height/2(Z)  "<Z>"
  height/1(U1) -> U1/1, operation/3(U1)
  Bus Selector1/2 -> "location "/4(Y)  "<Y>"
  Z_d/1 -> height/1(Z_d)
  Bus Selector1/1 -> "location "/3(X)  "<X>"
  Position/1 -> Bus Selector1/1
  "location "/2(Y') -> operation/2(Y')
  operation/2(Roll_d) -> Roll_d/1
  X_d/1 -> "location "/1(X_d)
  Y_d/1 -> "location "/2(Y_d)
  operation/1(Pitch_d) -> Pitch_d/1

== system Quadrotor/Quad_mathmodel ==
  U1 : Inport
  U2 : Inport  Port=2
  U3 : Inport  Port=3
  U4 : Inport  Port=4
  Euler system : Subsystem
      settings: PortSchema="{\"entries\":[{\"content\":{\"sides\":[{\"content\":{\"connectorIds\":[\"In1\",\"In2\",\"In3\",\"In4\"]},\"type\":\"ConnectorPlacement.EquallySpacedRectSide\",\"uuid\":\"24e9f502-01e2-4796-81d1-4356e5613cd4\"},{\"content\":{\"connectorIds\":[\"Out1\",\"Out2\",\"Out3\"],\"side\":\"RIGHT\"},\"type\":\"ConnectorPlacement.EquallySpacedRectSide\",\"uuid\":\"86fc2a55-a1b7-4625-a7fd-97b1845c6b1e\"},{\"content\":{\"connectorIds\":[],\"side\":\"TOP\"},\"type\":\"ConnectorPlacement.EquallySpacedRectSide\",\"uuid\":\"58e97d03-eced-4c7d-922b-6a4463cc6835\"},{\"content\":{\"connectorIds\":[\"In5\",\"In6\",\"In7\"],\"side\":\"BOTTOM\"},\"type\":\"ConnectorPlacement.EquallySpacedRectSide\",\"uuid\":\"f911275b-2fff-4eb0-817b-81b694121986\"}]},\"type\":\"ConnectorPlacement.EquallySpacedConnector\",\"uuid\":\"11616862-190a-491d-8e6d-3b18839a1b83\"}],\"packageUris\":[\"http://schema.mathworks.com/mf0/Connector/R2020b\"],\"version\":\"1.0\"}"
  Omega system : Subsystem
  Position system : Subsystem
      settings: PortSchema="{\"entries\":[{\"content\":{\"sides\":[{\"content\":{\"connectorIds\":[\"In1\",\"In2\",\"In3\",\"In4\"]},\"type\":\"ConnectorPlacement.EquallySpacedRectSide\",\"uuid\":\"4e608076-d82c-49dd-b9c3-40de08b530f0\"},{\"content\":{\"connectorIds\":[\"Out1\",\"Out2\",\"Out3\",\"Out4\",\"Out5\",\"Out6\"],\"side\":\"RIGHT\"},\"type\":\"ConnectorPlacement.EquallySpacedRectSide\",\"uuid\":\"79b98a7d-b351-461d-bf57-6a86461ab0e9\"},{\"content\":{\"connectorIds\":[],\"side\":\"TOP\"},\"type\":\"ConnectorPlacement.EquallySpacedRectSide\",\"uuid\":\"a0272396-a878-4308-9d2f-e99a972ffebc\"},{\"content\":{\"connectorIds\":[\"Out7\",\"Out8\",\"Out9\"],\"side\":\"BOTTOM\"},\"type\":\"ConnectorPlacement.EquallySpacedRectSide\",\"uuid\":\"679361ac-afba-4ea2-980e-22b3bd722f7e\"}]},\"type\":\"ConnectorPlacement.EquallySpacedConnector\",\"uuid\":\"cd6e232c-b153-4628-a51e-54595ea92055\"}],\"packageUris\":[\"http://schema.mathworks.com/mf0/Connector/R2020b\"],\"version\":\"1.0\"}"
  X : Outport
  Y : Outport  Port=2
  Z : Outport  Port=3
  Roll : Outport  Port=4
  Pitch : Outport  Port=5
  Yaw : Outport  Port=6
  wires:
  Position system/6(Yaw) -> Yaw/1
  Omega system/5(Omega) -> Euler system/4(Omega)
  Omega system/2(U2^2) -> Euler system/1(U2^2)
  Omega system/3(U3^2) -> Euler system/2(U3^2)
  Position system/2(Y) -> Y/1
  Omega system/1(U1^2) -> Position system/1(U1^2)
  Euler system/2(Pintch_dot_dot) -> Position system/3(Pintch_dot_dot)
  Omega system/4(U4^2) -> Euler system/3(U4^2)
  U3/1 -> Omega system/3(U3)
  Euler system/1(Roll_dot_dot) -> Position system/2(Roll_dot_dot)
  Euler system/3(Yaw_dot_dot) -> Position system/4(Yaw_dot_dot)
  Position system/3(Z) -> Z/1
  U1/1 -> Omega system/1(U1)
  Position system/4(Roll) -> Roll/1
  Position system/5(Pitch) -> Pitch/1
  Position system/1(X) -> X/1
  U2/1 -> Omega system/2(U2)
  U4/1 -> Omega system/4(U4)
  Position system/9(Roll_dot) -> Euler system/7(Roll_dot)
  Position system/8(Pintch_dot) -> Euler system/6(Pintch_dot)
  Position system/7(Yaw_dot) -> Euler system/5(Yaw_dot)

== system Quadrotor/Quadrotor_mathmodel ==
  U1 : Inport
  U2 : Inport  Port=2
  U3 : Inport  Port=3
  U4 : Inport  Port=4
  Euler system : Subsystem
      settings: PortSchema="{\"entries\":[{\"content\":{\"sides\":[{\"content\":{\"connectorIds\":[\"In1\",\"In2\",\"In3\",\"In4\"]},\"type\":\"ConnectorPlacement.EquallySpacedRectSide\",\"uuid\":\"24e9f502-01e2-4796-81d1-4356e5613cd4\"},{\"content\":{\"connectorIds\":[\"Out1\",\"Out2\",\"Out3\"],\"side\":\"RIGHT\"},\"type\":\"ConnectorPlacement.EquallySpacedRectSide\",\"uuid\":\"86fc2a55-a1b7-4625-a7fd-97b1845c6b1e\"},{\"content\":{\"connectorIds\":[],\"side\":\"TOP\"},\"type\":\"ConnectorPlacement.EquallySpacedRectSide\",\"uuid\":\"58e97d03-eced-4c7d-922b-6a4463cc6835\"},{\"content\":{\"connectorIds\":[\"In5\",\"In6\",\"In7\"],\"side\":\"BOTTOM\"},\"type\":\"ConnectorPlacement.EquallySpacedRectSide\",\"uuid\":\"f911275b-2fff-4eb0-817b-81b694121986\"}]},\"type\":\"ConnectorPlacement.EquallySpacedConnector\",\"uuid\":\"11616862-190a-491d-8e6d-3b18839a1b83\"}],\"packageUris\":[\"http://schema.mathworks.com/mf0/Connector/R2020b\"],\"version\":\"1.0\"}"
  Omega system : Subsystem
  Position system : Subsystem
      settings: PortSchema="{\"entries\":[{\"content\":{\"sides\":[{\"content\":{\"connectorIds\":[\"In1\",\"In2\",\"In3\",\"In4\"]},\"type\":\"ConnectorPlacement.EquallySpacedRectSide\",\"uuid\":\"4e608076-d82c-49dd-b9c3-40de08b530f0\"},{\"content\":{\"connectorIds\":[\"Out1\",\"Out2\",\"Out3\",\"Out4\",\"Out5\",\"Out6\"],\"side\":\"RIGHT\"},\"type\":\"ConnectorPlacement.EquallySpacedRectSide\",\"uuid\":\"79b98a7d-b351-461d-bf57-6a86461ab0e9\"},{\"content\":{\"connectorIds\":[],\"side\":\"TOP\"},\"type\":\"ConnectorPlacement.EquallySpacedRectSide\",\"uuid\":\"a0272396-a878-4308-9d2f-e99a972ffebc\"},{\"content\":{\"connectorIds\":[\"Out7\",\"Out8\",\"Out9\"],\"side\":\"BOTTOM\"},\"type\":\"ConnectorPlacement.EquallySpacedRectSide\",\"uuid\":\"679361ac-afba-4ea2-980e-22b3bd722f7e\"}]},\"type\":\"ConnectorPlacement.EquallySpacedConnector\",\"uuid\":\"cd6e232c-b153-4628-a51e-54595ea92055\"}],\"packageUris\":[\"http://schema.mathworks.com/mf0/Connector/R2020b\"],\"version\":\"1.0\"}"
  X : Outport
  Y : Outport  Port=2
  Z : Outport  Port=3
  Roll : Outport  Port=4
  Pitch : Outport  Port=5
  Yaw : Outport  Port=6
  wires:
  Position system/6(Yaw) -> Yaw/1
  Omega system/5(Omega) -> Euler system/4(Omega)
  Omega system/2(U2^2) -> Euler system/1(U2^2)
  Omega system/3(U3^2) -> Euler system/2(U3^2)
  Position system/2(Y) -> Y/1
  Omega system/1(U1^2) -> Position system/1(U1^2)
  Euler system/2(Pintch_dot_dot) -> Position system/3(Pintch_dot_dot)
  Omega system/4(U4^2) -> Euler system/3(U4^2)
  U3/1 -> Omega system/3(U3)
  Euler system/1(Roll_dot_dot) -> Position system/2(Roll_dot_dot)
  Euler system/3(Yaw_dot_dot) -> Position system/4(Yaw_dot_dot)
  Position system/3(Z) -> Z/1
  U1/1 -> Omega system/1(U1)
  Position system/4(Roll) -> Roll/1
  Position system/5(Pitch) -> Pitch/1
  Position system/1(X) -> X/1
  U2/1 -> Omega system/2(U2)
  U4/1 -> Omega system/4(U4)
  Position system/9(Roll_dot) -> Euler system/7(Roll_dot)
  Position system/8(Pintch_dot) -> Euler system/6(Pintch_dot)
  Position system/7(Yaw_dot) -> Euler system/5(Yaw_dot)

== system Quadrotor/UGV1 ==
  x_d : Inport
  y_d : Inport  Port=2
  xd : Outport
  yd : Outport  Port=2
  wires:
  x_d/1 -> xd/1
  y_d/1 -> yd/1

== system Quadrotor/UGV2 ==
  x_d : Inport
  y_d : Inport  Port=2
  xd : Outport
  yd : Outport  Port=2
  wires:
  x_d/1 -> xd/1
  y_d/1 -> yd/1

== system Quadrotor/Attitude Loop(LADRC)/LADRC ==
  v0 : Inport
  LESO : Subsystem
      settings: PortSchema="{\"entries\":[{\"content\":{\"sides\":[{\"content\":{\"connectorIds\":[\"In1\"]},\"type\":\"ConnectorPlacement.EquallySpacedRectSide\",\"uuid\":\"29853f4c-4dde-4de5-ade1-1dc0b5f537cd\"},{\"content\":{\"connectorIds\":[\"Out1\",\"Out2\",\"Out3\"],\"side\":\"RIGHT\"},\"type\":\"ConnectorPlacement.EquallySpacedRectSide\",\"uuid\":\"f82e0ac0-07eb-4296-b691-afdbd004b121\"},{\"content\":{\"connectorIds\":[\"In2\"],\"side\":\"TOP\"},\"type\":\"ConnectorPlacement.EquallySpacedRectSide\",\"uuid\":\"058c0543-22b7-4f39-8eab-a4fe87266d7e\"}]},\"type\":\"ConnectorPlacement.EquallySpacedConnector\",\"uuid\":\"8c454db7-eb5f-43d2-ac3f-1394779a05da\"}],\"packageUris\":[\"http://schema.mathworks.com/mf0/Connector/19700101\"],\"version\":\"1.0\"}"
  LESO1 : Subsystem
      settings: PortSchema="{\"entries\":[{\"content\":{\"sides\":[{\"content\":{\"connectorIds\":[\"In1\"]},\"type\":\"ConnectorPlacement.EquallySpacedRectSide\",\"uuid\":\"29853f4c-4dde-4de5-ade1-1dc0b5f537cd\"},{\"content\":{\"connectorIds\":[\"Out1\",\"Out2\",\"Out3\"],\"side\":\"RIGHT\"},\"type\":\"ConnectorPlacement.EquallySpacedRectSide\",\"uuid\":\"f82e0ac0-07eb-4296-b691-afdbd004b121\"},{\"content\":{\"connectorIds\":[\"In2\"],\"side\":\"TOP\"},\"type\":\"ConnectorPlacement.EquallySpacedRectSide\",\"uuid\":\"058c0543-22b7-4f39-8eab-a4fe87266d7e\"}]},\"type\":\"ConnectorPlacement.EquallySpacedConnector\",\"uuid\":\"8c454db7-eb5f-43d2-ac3f-1394779a05da\"}],\"packageUris\":[\"http://schema.mathworks.com/mf0/Connector/19700101\"],\"version\":\"1.0\"}"
  LSEF : Subsystem
  LSEF1 : Subsystem
  Object : Subsystem
  Object1 : Subsystem
  Sum{,1..4} (5 alike) : Sum  Inputs=|+-
  TD : Subsystem
  b1 : Gain  Gain=b
  b2 : Gain  Gain=1/b
  b3 : Gain  Gain=1/b
  b4 : Gain  Gain=1/b
  y : Outport
  wires:
  LSEF/1(u0) -> Sum2/1
  Object/1(y) -> y/1, LESO/1(y)
  LESO/1(z3) -> Sum2/2
  Sum2/1 -> b2/1  "e1"
  b2/1 -> LESO/2(u), Object/1(u)
  Sum/1 -> LSEF/1(e1)  "e1"
  v0/1 -> Sum/1, TD/1(v0)
  LESO/3(z1) -> Sum/2  "z1"
  LESO/2(z2) -> LSEF/2(e2)  "z2"
  Object1/1(y) -> LESO1/1(y)
  LESO1/3(z1) -> Sum1/2  "z1"
  LSEF1/1(u0) -> Sum3/1
  Sum1/1 -> LSEF1/1(e1)  "e1"
  b3/1 -> Object1/1(u)
  Sum3/1 -> b3/1  "e1"
  LESO1/1(z3) -> Sum3/2
  TD/1(v1) -> Sum1/1
  LESO1/2(z2) -> Sum4/2  "z2"
  TD/2(v2) -> Sum4/1
  Sum4/1 -> LSEF1/2(e2)  "e1"

== system Quadrotor/Attitude Loop(LADRC)/LADRC1 ==
  v0 : Inport
  y : Inport  Port=2
  LESO : Subsystem
      settings: PortSchema="{\"entries\":[{\"content\":{\"sides\":[{\"content\":{\"connectorIds\":[]},\"type\":\"ConnectorPlacement.EquallySpacedRectSide\",\"uuid\":\"29853f4c-4dde-4de5-ade1-1dc0b5f537cd\"},{\"content\":{\"connectorIds\":[\"Out1\",\"Out2\",\"Out3\"],\"side\":\"RIGHT\"},\"type\":\"ConnectorPlacement.EquallySpacedRectSide\",\"uuid\":\"f82e0ac0-07eb-4296-b691-afdbd004b121\"},{\"content\":{\"connectorIds\":[\"In1\"],\"side\":\"TOP\"},\"type\":\"ConnectorPlacement.EquallySpacedRectSide\",\"uuid\":\"058c0543-22b7-4f39-8eab-a4fe87266d7e\"},{\"content\":{\"connectorIds\":[\"In2\"],\"side\":\"BOTTOM\"},\"type\":\"ConnectorPlacement.EquallySpacedRectSide\",\"uuid\":\"5206ee30-69dc-4d41-920c-ca25503196a3\"}]},\"type\":\"ConnectorPlacement.EquallySpacedConnector\",\"uuid\":\"8c454db7-eb5f-43d2-ac3f-1394779a05da\"}],\"packageUris\":[\"http://schema.mathworks.com/mf0/Connector/19700101\"],\"version\":\"1.0\"}"
  LSEF : Subsystem
  Sum : Sum  Inputs=|+-
  Sum2 : Sum  Inputs=|+-
  b2 : Gain  Gain=1/b
  u : Outport
  wires:
  LESO/3(z1) -> Sum/2  "z1"
  LSEF/1(u0) -> Sum2/1
  Sum/1 -> LSEF/1(e1)  "e1"
  v0/1 -> Sum/1
  LESO/2(z2) -> LSEF/2(e2)  "z2"
  LESO/1(z3) -> Sum2/2
  Sum2/1 -> b2/1  "e1"
  b2/1 -> u/1, LESO/1(u)
  y/1 -> LESO/2(y)

== system Quadrotor/Attitude Loop(LADRC)/P&R ==
  Pitch_d : Inport
  Roll_d : Inport  Port=2
  Pitch : Inport  Port=3
  Roll : Inport  Port=4
  Pitch_LADRC : Subsystem  mask{h=0.0005, r=10, beta01=90, beta02=2700, beta03=27000, kp1=80, kp2=20, b=30}
      mask DialogControl ParameterGroupVar Prompt: 四旋翼参数
      mask DialogControl Container3 Prompt: 步长
      mask DialogControl Container4 Prompt: 跟踪速度
      mask DialogControl Container5 Prompt: 增益
      mask DialogControl Container6 Prompt: 系统增益
  Roll_LADRC : Subsystem  mask{h=0.0005, r=10, beta01=90, beta02=2700, beta03=27000, kp1=80, kp2=20, b=30}
      mask DialogControl ParameterGroupVar Prompt: 四旋翼参数
      mask DialogControl Container3 Prompt: 步长
      mask DialogControl Container4 Prompt: 跟踪速度
      mask DialogControl Container5 Prompt: 增益
      mask DialogControl Container6 Prompt: 系统增益
  U3 : Outport
  U2 : Outport  Port=2
  wires:
  Roll_d/1 -> Roll_LADRC/1(v0)
  Roll/1 -> Roll_LADRC/2(y)
  Roll_LADRC/1(u) -> U2/1
  Pitch_LADRC/1(u) -> U3/1
  Pitch_d/1 -> Pitch_LADRC/1(v0)
  Pitch/1 -> Pitch_LADRC/2(y)

== system Quadrotor/Attitude Loop(LADRC)/yaw ==
  Yaw_d : Inport
  Yaw : Inport  Port=2
  Yaw_LADRC : Subsystem  mask{h=0.0005, r=10, beta01=30, beta02=100, beta03=1000, kp1=100, kp2=20, b=80}
      mask DialogControl ParameterGroupVar Prompt: 四旋翼参数
      mask DialogControl Container3 Prompt: 步长
      mask DialogControl Container4 Prompt: 跟踪速度
      mask DialogControl Container5 Prompt: 增益
      mask DialogControl Container6 Prompt: 系统增益
  U4 : Outport
  wires:
  Yaw/1 -> Yaw_LADRC/2(y)
  Yaw_d/1 -> Yaw_LADRC/1(v0)
  Yaw_LADRC/1(u) -> U4/1
